simulink model "Practica4"  (R2014b)
settings: Solver=ode45  StartTime=0.0  StopTime=100  RelTol=1e-3
libraries: fuzblock x1
settings Model: Creator=usuario_local  LastModifiedBy=usuario_local

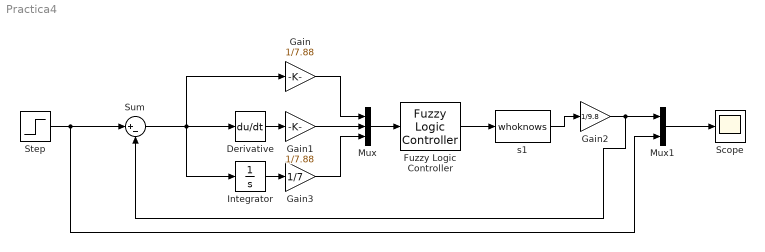
== system Practica4 ==
  Derivative : Derivative
  Fuzzy Logic Controller : fuzblock/Fuzzy Logic  Controller  fis='FuzzyControllerPIDv4.fis'
  Gain : Gain  Gain=1/7.88
  Gain1 : Gain  Gain=1/7.88
  Gain2 : Gain  Gain=1/9.8
  Gain3 : Gain  Gain=1/7
  Integrator : Integrator
  Mux : Mux  Inputs=3
  Mux1 : Mux  Inputs=2
  Scope : Scope
      settings: TimeRange=100  YMin=0  YMax=1.2
  Step : Step  SampleTime=0  ZeroCross=off
  Sum : Sum  Inputs=|+-
  s1 : M-S-Function  FunctionName=whoknows  Parameters=L, P1, P2, T, R  mask{L=6, P1=0, P2=3, T=1, R=0}
      mask prompts: L "Laboratorio"; P1 "Primer digito del Puesto"; P2 "Segundo digito del Puesto"; T "Tipo de Planta"; R "Ruido"
      mask Display: disp('Sistema')
  wires:
  Step/1 -> Mux1/2, Sum/1
  Sum/1 -> Integrator/1, Gain/1, Derivative/1
  Fuzzy Logic Controller/1 -> s1/1
  Mux1/1 -> Scope/1
  Derivative/1 -> Gain1/1
  s1/1 -> Gain2/1
  Gain2/1 -> Sum/2, Mux1/1
  Integrator/1 -> Gain3/1
  Mux/1 -> Fuzzy Logic Controller/1
  Gain/1 -> Mux/1
  Gain1/1 -> Mux/2
  Gain3/1 -> Mux/3
